simulink library "cdsEpicsOut"  (Simulink 6.2)
settings Model: LastModifiedBy=rolf

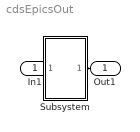
== system cdsEpicsOut ==
  In1 : Inport  Port=1  LatchInput=off
  Subsystem : Subsystem
  Out1 : Outport
  wires:
  Subsystem/1(Out1) -> Out1/1
  In1/1 -> Subsystem/1(In1)

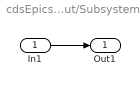
== system cdsEpicsOut/Subsystem ==
  In1 : Inport  Port=1  LatchInput=off
  Out1 : Outport
  wires:
  In1/1 -> Out1/1
